simulink model "FreePortComm_RX_7Seg_MiniDragon"  (Simulink 7.4)
settings: Solver=FixedStepDiscrete  SolverMode=SingleTasking  StartTime=0.0  StopTime=inf  FixedStep=.02  RelTol=1e-3
settings Model: Creator=fwornle  LastModifiedBy=fw  SimulationMode=external  ExtModeTrigDuration=500
settings ConfigSet: Description=rtmc9s12target_R2009b
settings DataIOCC: SignalLoggingName=sigsOut
settings OptimizationCC: BooleanDataType=off  InitFltsAndDblsToZero=on  OptimizeModelRefInitCode=on  LifeSpan=1
settings DebuggingCC: SaveWithParameterizedLinksMsg=none  SignalResolutionControl=TryResolveAllWithWarning  SolverPrmCheckMsg=none  MultiTaskDSMMsg=warning  MultiTaskCondExecSysMsg=none  StrictBusMsg=None
settings HardwareCC: ProdBitPerInt=16  ProdEndianess=BigEndian  ProdWordSize=16  ProdHWDeviceType=Motorola HC12
settings RTWCC: SystemTargetFile=mc9s12.tlc  GenerateMakefile=off  TemplateMakefile=mc9s12.tmf  ProcessScript=mc9s12_make_rtw_hook  IncludeERTFirstTime=on
settings CodeAppCC: IgnoreCustomStorageClasses=off
settings STFCustomTargetCC: TargetFcnLib=ansi_tfl_tmw.mat  ModelReferenceCompliant=off  IncludeMdlTerminateFcn=off  ERTCustomFileBanners=on  SupportNonInlinedSFcns=off  CPPClassGenCompliant=on  SystemTargetFile=mc9s12.tlc
settings ERTTargetCC: TargetFcnLib=ansi_tfl_tmw.mat  MultiwordLength=2048  ModelReferenceCompliant=off  ParMdlRefBuildCompliant=off  CompOptLevelCompliant=off  IncludeMdlTerminateFcn=off  CombineOutputUpdateFcns=off  ERTFirstTimeCompliant=off  SupportContinuousTime=on  ModelStepFunctionPrototypeControlCompliant=off  ExtMode=on  ExtModeMexFile=ext_serial_mc9s12_comm  ExtModeMexArgs=1,2,115200  InlinedParameterPlacement=NonHierarchical  ERTCustomFileTemplate=mc9s12_file_process.tlc  GRTInterface=on  ConvertIfToSwitch=off
settings CustomProperty: DataType=RTWOptions_EnumType_C__Users_fw__SVN_rtmc9s12-target_trunk_rtmc9s12_CW_R2009b_bin_mc9s12_1mc9s12_TargetBoard  Value=Dragon12Plus
settings EnumStrPairs: String=Dragon12

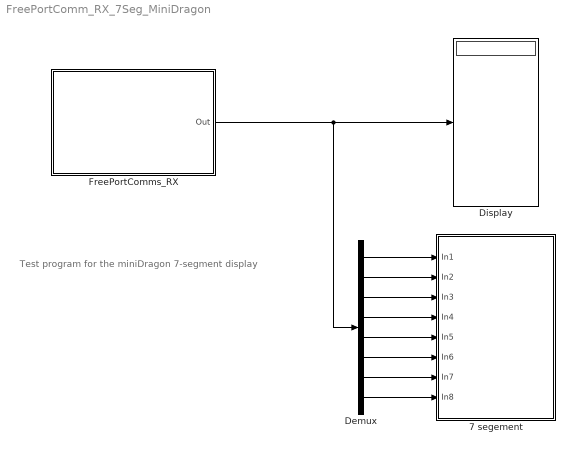
== system FreePortComm_RX_7Seg_MiniDragon ==
  note: Test program for the
      | miniDragon 7-segment display
  7 segement : Subsystem  Tag=mcTarget_digOut  mask{port=Port H, pin=0 1 2 3 4 5 6 7, sampletime=0.02, Von=0.5, Voff=0.5}
      mask prompts: port "Port (see hardware manuals for valid options)"; pin "Pin (see hardware manuals for valid options)"; sampletime "Sample time"; Von "On-threshold (Von)"; Voff "Off-threshold (Voff)"
      mask init:
      | [portstr, pinstr, pins] = mbc_digitaloutput(port, pin, sampletime, Von, Voff);
      mask Help: web('digOut_sfcn_9S12.html');
      mask StyleString: popup(Port A|Port B|Port H|Port J|Port M|Port P|Port S|Port T),edit,edit,edit,edit
      mask Display: fprintf('%s\nPins: %s', portstr, pinstr)
  Demux : Demux  Outputs=8
  Display : Display
  FreePortComms_RX : Subsystem  Tag=mcTarget_freePortCommsRX  mask{sampletime=0.1, port=SCI0, baudrate=115200, channel=0, buf_size=8, data_type=UINT8, format=off, outformat=on}
      mask prompts: sampletime "Sample time"; port "Communication port"; channel "Channel number"; buf_size "Number of elements"; data_type "Data Type"; format "Block receives raw data"; outformat "Block output is double"
      mask init:
      | [buf_sizestr, portNamestr, baudratestr, channelstr, data_type_str, sampletime_str] = mbc_freeportrxd(sampletime, port, baudrate, channel, buf_size, data_type, format, outformat);
      mask Help: web('freePortComms_rxd.html');
      mask StyleString: edit,popup(SCI0|SCI1|COM1|COM2|COM3|COM4),popup(300|600|1200|2400|4800|9600|19200|38400|57600|115200),edit,edit,popup(SINGLE|INT8|UINT8|INT16|UINT16|INT32|UINT32|BOOLEAN),checkbox,checkbox
      mask Display: fprintf('Receive %s element(s)\nComm port: %s\nBaudrate: %s bps\nChannel: %s\nData type: %s\n Sample rate: %s', buf_sizestr, portNamestr, baudratestr, channelstr, data_type_str, sampletime_str)
  wires:
  FreePortComms_RX/1(Out) -> Display/1, Demux/1
  Demux/1 -> 7 segement/1(In1)
  Demux/2 -> 7 segement/2(In2)
  Demux/3 -> 7 segement/3(In3)
  Demux/4 -> 7 segement/4(In4)
  Demux/5 -> 7 segement/5(In5)
  Demux/6 -> 7 segement/6(In6)
  Demux/7 -> 7 segement/7(In7)
  Demux/8 -> 7 segement/8(In8)

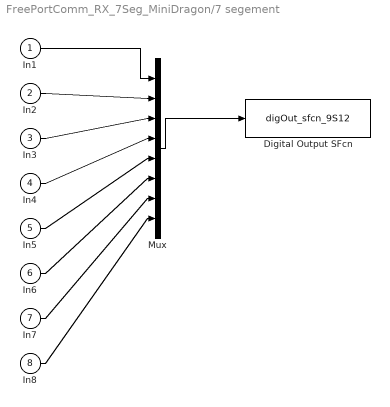
== system FreePortComm_RX_7Seg_MiniDragon/7 segement ==
  In1 : Inport  OutDataType=sfix(16)  OutScaling=2^0
  In2 : Inport  Port=2  OutDataType=sfix(16)  OutScaling=2^0
  In3 : Inport  Port=3  OutDataType=sfix(16)  OutScaling=2^0
  In4 : Inport  Port=4  OutDataType=sfix(16)  OutScaling=2^0
  In5 : Inport  Port=5  OutDataType=sfix(16)  OutScaling=2^0
  In6 : Inport  Port=6  OutDataType=sfix(16)  OutScaling=2^0
  In7 : Inport  Port=7  OutDataType=sfix(16)  OutScaling=2^0
  In8 : Inport  Port=8  OutDataType=sfix(16)  OutScaling=2^0
  Digital Output SFcn : S-Function  Tag=mcTarget_digOut  FunctionName=digOut_sfcn_9S12  Parameters=sampletime, port, pins, Von, Voff  EnableBusSupport=off
  Mux : Mux  Inputs=8
  wires:
  Mux/1 -> Digital Output SFcn/1
  In1/1 -> Mux/1
  In2/1 -> Mux/2
  In3/1 -> Mux/3
  In4/1 -> Mux/4
  In5/1 -> Mux/5
  In6/1 -> Mux/6
  In7/1 -> Mux/7
  In8/1 -> Mux/8

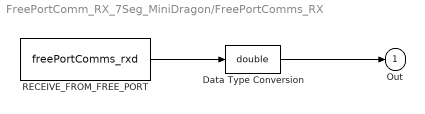
== system FreePortComm_RX_7Seg_MiniDragon/FreePortComms_RX ==
  Data Type Conversion : DataTypeConversion  OutDataTypeMode=double  OutDataType=sfix(16)  OutScaling=2^0  OutDataTypeStr=double  SaturateOnIntegerOverflow=on  RndMeth=Zero
  RECEIVE_FROM_FREE_PORT : S-Function  Tag=mcTarget_freePortCommsRX  FunctionName=freePortComms_rxd  Parameters=sampletime, channel, buf_size, data_type, port, baudrate, format  EnableBusSupport=off
  Out : Outport  OutDataType=sfix(16)  OutScaling=2^0
  wires:
  RECEIVE_FROM_FREE_PORT/1 -> Data Type Conversion/1
  Data Type Conversion/1 -> Out/1
